simulink model "Part3_1"  (R2021b)
settings: Solver=VariableStepAuto  StartTime=0.0  StopTime=10.0  RelTol=1e-3
settings Model: Creator=Matin  LastModifiedBy=Matin

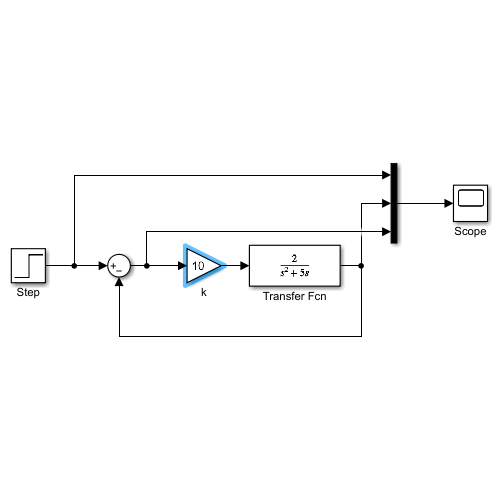
[thumbnail: Simulink's stored preview of the top-level diagram]
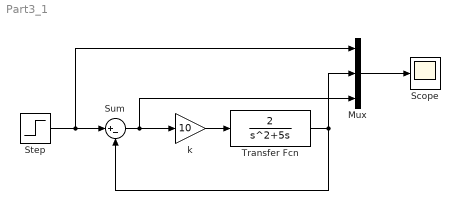
== system Part3_1 ==
  Mux : Mux  Inputs=3
  Scope : Scope
  Step : Step  SampleTime=0
  Sum : Sum  Inputs=|+-
  Transfer Fcn : TransferFcn  Numerator=[2]  Denominator=[1 5 0]
  k : Gain  Gain=10
  wires:
  Step/1 -> Sum/1, Mux/1
  k/1 -> Transfer Fcn/1
  Transfer Fcn/1 -> Mux/2, Sum/2
  Mux/1 -> Scope/1
  Sum/1 -> Mux/3, k/1
